simulink model "HESS_PassiveModel"  (R2018b)
settings: Solver=VariableStepAuto  StartTime=0.0  StopTime=1400  MaxStep=0.01  MinStep=0.00005  RelTol=1e-3
undefined symbols (not defined in the file or in its folder): Ion, Lithium
libraries: powerlib x5, electricdrivelib x2
settings Model: Creator=ttran  LastModifiedBy=ttran
settings SolverCC: ZeroCrossControl=EnableAll
settings DebuggingCC: IgnoredZcDiagnostic=none  SolverPrmCheckMsg=warning

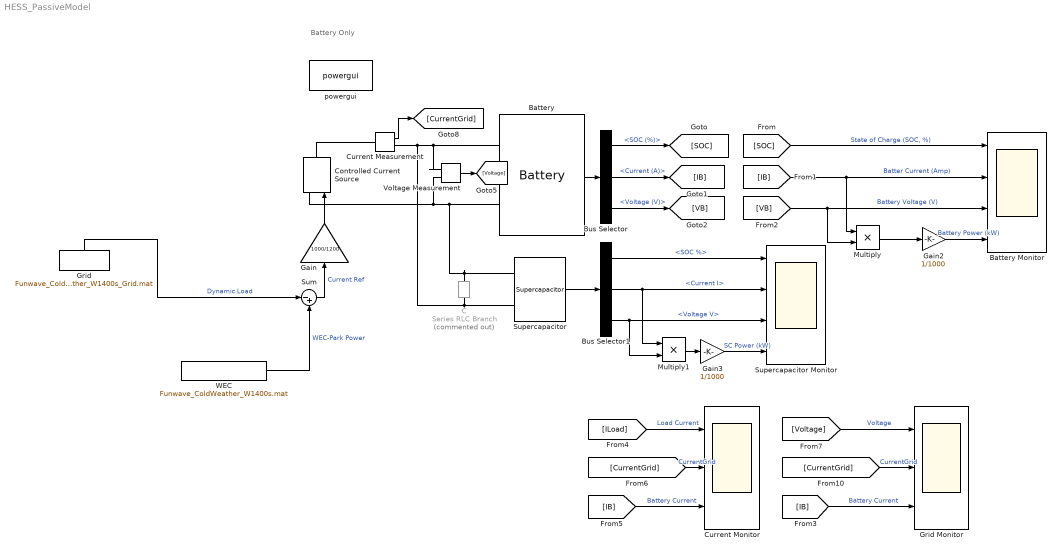
== system HESS_PassiveModel ==
  note: Battery Only
  Battery : electricdrivelib/Extra Sources/Battery  BatType=Lithium-Ion  ShowTempParam=off  ThermalPreset=no  ShowAgeParam=off  NomV=340  NomQ=73  SOC=50  Batt_Tr=1e-4  PresetModel=on  MaxQ=73  MinV=255  FullV=395.7556  Dis_rate=31.7391  R=0.046575  Normal_OP=66.0174  expZone="[367.3312      3.586522]"  current=[6.5 13 32.5]  Units=Time  Tci=20  NomT=20  T2=-30  MaxQ2=4.8  FullV2=7.1  Normal_OP2=5.655  expZone2="[6.58           1]"  Rca=0.6  ti=2000  Dp=0  Neq0=0  Tsim=1e6  Ta1=25  Qeol=5.4*0.9  Reol=0.013333*1.2  Char_age=[2.3478, 3]  Dis_age=[2.3478, 10]  N1=1500  N2=10500  N3=1000  N4=1400  Ta2=45  N5=950
  Battery Monitor : Scope  NumInputPorts=4
  Bus Selector : BusSelector  OutputSignals=SOC (%),Current (A),Voltage (V)
  Bus Selector1 : BusSelector  OutputSignals=SOC %,Current I,Voltage V
  C : powerlib/Elements/Series RLC Branch  Commented=on  LConnTagsString=__new0  RConnTagsString=__new0  BranchType=C  Resistance=1  Inductance=1e-3  SetiL0=off  InitialCurrent=0  Capacitance=0.1  Setx0=off  InitialVoltage=0  Measurements=None
  Controlled Current Source : powerlib/Electrical Sources/Controlled Current Source  Initialize=on  Source_Type=AC  Amplitude=0  Phase=0  Frequency=0  Measurements=None
  Current Measurement : powerlib/Measurements/Current Measurement  PhasorSimulation=off  OutputType=Complex  PSBequivalent=0
  Current Monitor : Scope  NumInputPorts=3
  Gain : Gain  Gain=1000/1200
  Gain2 : Gain  Gain=1/1000
  Gain3 : Gain  Gain=1/1000
  Grid : FromFile  FileName=Funwave_ColdWeather_W1400s_Grid.mat  SampleTime=0
  Grid Monitor : Scope  NumInputPorts=3
  Multiply : Product
  Multiply1 : Product
  Sum : Sum  Inputs=|-+
  Supercapacitor : electricdrivelib/Extra Sources/Supercapacitor  C=760  Rdc=8.9e-3  Voltage=380  Ns=144  Np=1  Vinit=340  Temp=25  PresetModel=off  EstParam=off  Nc=1  r=1e-9  epsilon=6.0208e-10  Ich=10  Vstern="[0.161  2.7  7.8]"  Self_dis=on  Ioc=10  Vself="[48  47.8  47.06  44.65]"  demandeplot=off  I="[10  20 100  500]"  Units=sec  Vmax=0  If=0  deltaV=0  alpha=0  sec=0
      settings: SourceProductName=Simscape Power Systems  SourceProductBaseCode=PS
  Supercapacitor Monitor : Scope  NumInputPorts=4
  Voltage Measurement : powerlib/Measurements/Voltage Measurement  PhasorSimulation=off  OutputType=Complex  PSBequivalent=0
  WEC : FromFile  FileName=Funwave_ColdWeather_W1400s.mat  SampleTime=0
  powergui : powerlib/powergui  Priority=1  SimulationMode=Continuous  SampleTime=50e-6  frequency=60  Iterations=50  frequencyindice=0  Pbase=100e6  ErrMax=1e-4  UnitsV=kV  UnitsW=MW  buscounter=0  FunctionMessages=off  echomessages=off  EnableUseOfTLC=off  CurrentSourceSwitches=off  DisableSnubberDevices=off  DisableRonSwitches=off  DisableVfSwitches=off  DisplayEquations=off  SolverType=Tustin/Backward Euler (TBE)  Interpol=off  ExternalGateDelay=off  methode=off  Ts=100  x0status=blocks  SPID=on  SwTol=0  HookPort=off  RestoreLinks=warning  ResistiveCurrentMeasurement=off  Frange=[0:2:500]  Ylog=off  Xlog=on  ShowGrid=off  save=off  variable=ZData  structure=0  ZoomFFT=off  StartTime=0.0  cycles=1  DisplayStyle=1  fundamental=60  FreqAxis=off  MaxFrequency=1000  frequencyindicesteady=1  RmsSteady=1  display=off
  wires:
  Battery/1 -> Bus Selector/1
  Bus Selector/1 -> [SOC]  "<SOC (%)>"
  Bus Selector/2 -> [IB]  "<Current (A)>"
  Bus Selector/3 -> [VB]  "<Voltage (V)>"
  [SOC] -> Battery Monitor/1  "State of Charge (SOC, %)"
  [IB] -> Battery Monitor/2, Multiply/1  "Batter Current (Amp)"
  [VB] -> Multiply/2, Battery Monitor/3  "Battery Voltage (V)"
  Multiply/1 -> Gain2/1
  Voltage Measurement/1 -> [Voltage]
  [Voltage] -> Grid Monitor/1  "Voltage"
  Current Measurement/1 -> [CurrentGrid]
  [CurrentGrid] -> Grid Monitor/2  "CurrentGrid"
  [IB] -> Grid Monitor/3  "Battery Current"
  Grid/1 -> Sum/1  "Dynamic Load"
  [IB] -> Current Monitor/3  "Battery Current"
  [ILoad] -> Current Monitor/1  "Load Current"
  [CurrentGrid] -> Current Monitor/2  "CurrentGrid"
  Bus Selector1/1 -> Supercapacitor Monitor/1  "<SOC %>"
  Bus Selector1/2 -> Supercapacitor Monitor/2, Multiply1/1  "<Current I>"
  Bus Selector1/3 -> Supercapacitor Monitor/3, Multiply1/2  "<Voltage V>"
  Multiply1/1 -> Gain3/1
  Supercapacitor/1 -> Bus Selector1/1
  Gain2/1 -> Battery Monitor/4  "Battery Power (kW)"
  Gain3/1 -> Supercapacitor Monitor/4  "SC Power (kW)"
  WEC/1 -> Sum/2  "WEC-Park Power"
  Gain/1 -> Controlled Current Source/1
  Sum/1 -> Gain/1  "Current Ref"
  connections:
  Supercapacitor/LConn2 -- C/LConn1 -- Battery/LConn2 -- Controlled Current Source/LConn1 -- Voltage Measurement/LConn2
  Current Measurement/LConn1 -- Controlled Current Source/RConn1
  Voltage Measurement/LConn1 -- Supercapacitor/LConn1 -- C/RConn1 -- Current Measurement/RConn1 -- Battery/LConn1
